simulink model "sunVector_test"  (R2018b)
settings: Solver=VariableStepAuto  StartTime=0.0  StopTime=0  RelTol=1e-3
values from neighbouring files (symbols this model uses):
  utc_test = 137803367    [solarPressure_test_init.m]    (also in sunVector_test_init.m = 197208000)
libraries: sunVector_lib x1, time_Lib x1
settings Model: Creator=devantormey  LastModifiedBy=devantormey

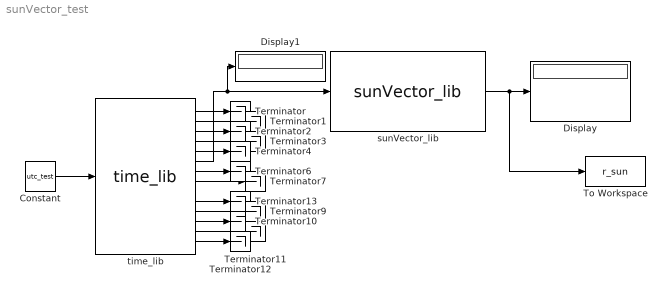
== system sunVector_test ==
  Constant : Constant  Value=utc_test
  Display : Display
  Display1 : Display
  Terminator{,1..4,6..7,9..13} (12 alike) : Terminator
  To Workspace : ToWorkspace  VariableName=r_sun  SaveFormat=Timeseries  SampleTime=-1
  sunVector_lib : sunVector_lib/sunVector_lib  SystemSampleTime=-1
  "time_lib " : time_Lib/time_lib    SystemSampleTime=-1
  wires:
  "time_lib "/3 -> Terminator2/1
  "time_lib "/12 -> Terminator10/1
  "time_lib "/5 -> Terminator4/1
  "time_lib "/2 -> Terminator1/1
  "time_lib "/4 -> Terminator3/1
  "time_lib "/13 -> Terminator11/1
  "time_lib "/11 -> Terminator9/1
  "time_lib "/7 -> Terminator6/1
  "time_lib "/8 -> Terminator7/1
  "time_lib "/1 -> Terminator/1
  "time_lib "/14 -> Terminator12/1
  sunVector_lib/1 -> To Workspace/1, Display/1
  "time_lib "/10 -> Terminator13/1
  Constant/1 -> "time_lib "/1
  "time_lib "/6 -> Display1/1, sunVector_lib/1
